simulink model "simrewinder_scaled_dig"  (R2023a)
settings: Solver=FixedStepDiscrete  StartTime=0.0  StopTime=200  FixedStep=ts  RelTol=1e-3
values from neighbouring files (symbols this model uses):
  b = alpha*(a+Kt*Kv)    [outperpi.m]
  Keg = egv/egz    (= 3149.60629921)    [outperpi.m]
  Kl = 8/0.1    (= 80)    [outperpi.m]
  Kp = Kpmax*10^(log10(wc/wmax))    [outperpi.m]
  Td = 0    [outperpi.m]
  umax = 5    [outperpi.m]
undefined symbols (not defined in the file or in its folder): dend, DiscIntNeverNeededParam, numd
settings Model: Creator=mike_  LastModifiedBy=mike_
settings DataIOCC: ReturnWorkspaceOutputs=off
settings DebuggingCC: UnconnectedInputMsg=warning  UnconnectedOutputMsg=warning  UnconnectedLineMsg=warning
settings ModelReferenceCC: EnableRefExpFcnMdlSchedulingChecks=on
settings RTWCC: DLArmComputeVersion=19.05

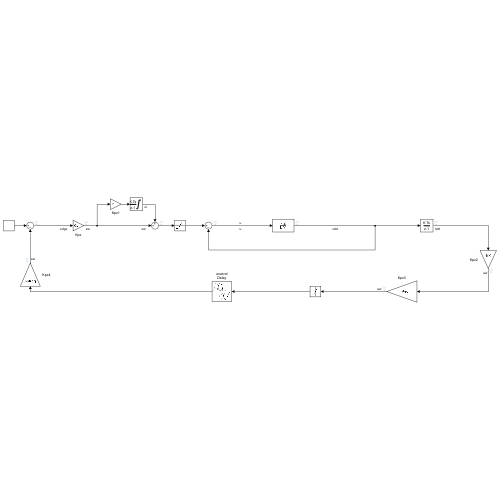
[thumbnail: Simulink's stored preview of the top-level diagram]
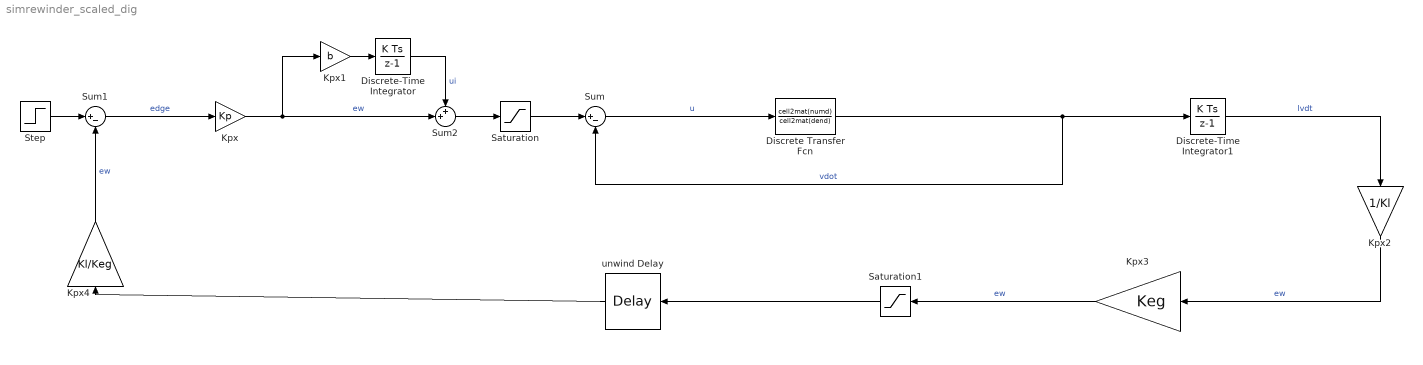
== system simrewinder_scaled_dig ==
  Discrete Transfer Fcn : DiscreteTransferFcn  Numerator=cell2mat(numd)  Denominator=cell2mat(dend)
  Discrete-Time Integrator : DiscreteIntegrator  SampleTime=-1  LimitOutput=on  UpperSaturationLimit=umax  LowerSaturationLimit=-umax  ICPrevOutput=DiscIntNeverNeededParam  ICPrevScaledInput=DiscIntNeverNeededParam
  Discrete-Time Integrator1 : DiscreteIntegrator  SampleTime=-1  ICPrevOutput=DiscIntNeverNeededParam  ICPrevScaledInput=DiscIntNeverNeededParam
  Kpx : Gain  Gain=Kp
  Kpx1 : Gain  Gain=b
  Kpx2 : Gain  Gain=1/Kl
  Kpx3 : Gain  Gain=Keg
  Kpx4 : Gain  Gain=Kl/Keg
  Saturation : Saturate  UpperLimit=umax  LowerLimit=-umax
  Saturation1 : Saturate  UpperLimit=10  LowerLimit=-10
  Step : Step  Time=2  After=.08  SampleTime=0
  Sum : Sum  Inputs=|+-
  Sum1 : Sum  Inputs=|+-
  Sum2 : Sum  Inputs=++|
  unwind Delay : TransportDelay  DelayTime=Td
  wires:
  Discrete Transfer Fcn/1 -> Discrete-Time Integrator1/1, Sum/2  "vdot"
  Step/1 -> Sum1/1
  unwind Delay/1 -> Kpx4/1
  Discrete-Time Integrator1/1 -> Kpx2/1  "lvdt"
  Sum/1 -> Discrete Transfer Fcn/1  "u"
  Sum2/1 -> Saturation/1
  Kpx1/1 -> Discrete-Time Integrator/1
  Discrete-Time Integrator/1 -> Sum2/1  "ui"
  Kpx/1 -> Sum2/2, Kpx1/1  "ew"
  Saturation/1 -> Sum/1
  Kpx2/1 -> Kpx3/1  "ew"
  Sum1/1 -> Kpx/1  "edge"
  Kpx4/1 -> Sum1/2  "ew"
  Kpx3/1 -> Saturation1/1  "ew"
  Saturation1/1 -> unwind Delay/1
